simulink subsystem "Human_Input_Pre_Processing"  (R2023b)
settings: Solver=VariableStepAuto  StartTime=0.0  StopTime=10.0  RelTol=1e-3
undefined symbols (not defined in the file): Gamepad_Stick_Neg_Threshold, Gamepad_Stick_Pos_Threshold, Test_DC_Gain_BackLower, Test_DC_Gain_BackUpper, Test_DC_Gain_BallScrew, Test_DC_Gain_Front, Test_DC_Gain_Intake, Test_DC_Gain_Shooter
libraries: simulink x28
settings Model: Creator=ander  LastModifiedBy=ander

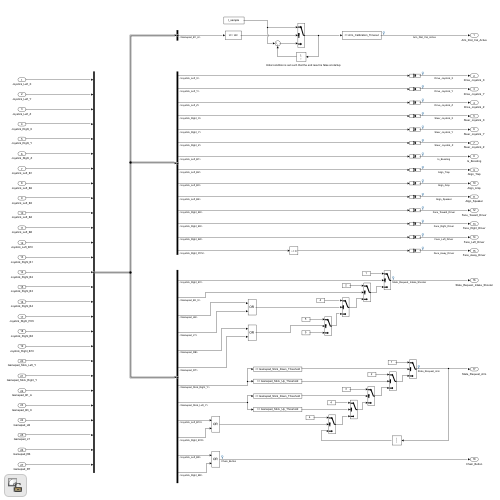
[thumbnail: Simulink's stored preview of the top-level diagram]
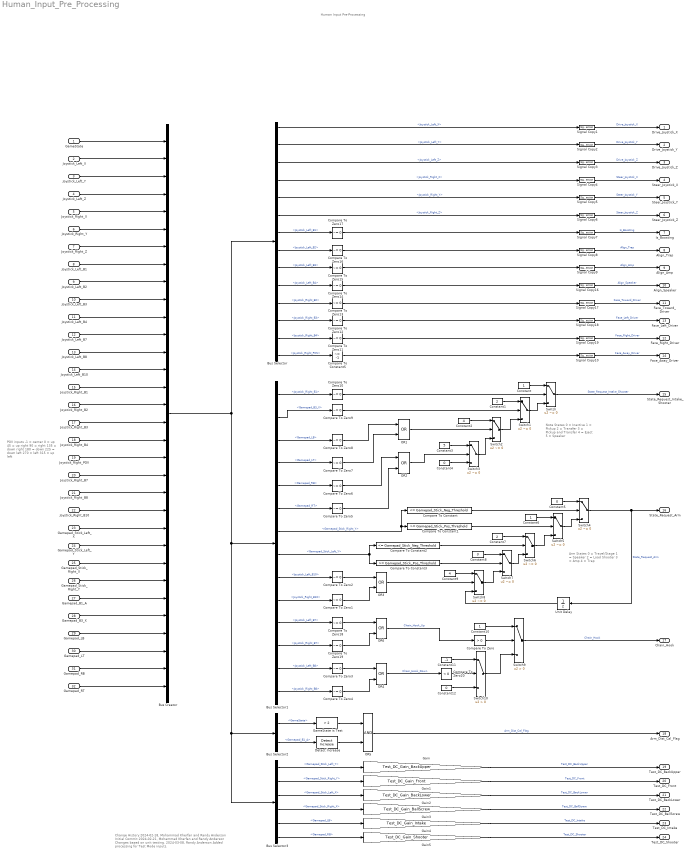
== system Human_Input_Pre_Processing ==
  note: POV inputs
      | -1 = center
      | 0 = up
      | 45 = up right
      | 90 = right
      | 135 = down right
      | 180 = down
      | 225 = down left
      | 270 = left
      | 315 = up left
  note: Human Input Pre-Processing
  note: Change History
      | 2024-02-18, Mohammad Kherfan and Randy Anderson
      | Initial Commit
      | 2024-02-21, Mohammad Kherfan and Randy Anderson
      | Changes based on unit testing.
      | 2024-03-08, Randy Anderson
      | Added processing for Test Mode inputs.
  note: Arm States
      | 0 = Travel/Stage
      | 1 = Speaker
      | 2 = Load Shooter
      | 3 = Amp
      | 4 = Trap
  note: Note States
      | 0 = Inactive
      | 1 = Pickup
      | 2 = Transfer
      | 3 = Pickup and Transfer
      | 4 = Eject
      | 5 = Speaker
  GameState : Inport
  Joystick_Left_X : Inport  Port=2
  Joystick_Left_Y : Inport  Port=3
  Joystick_Left_Z : Inport  Port=4
  Joystick_Right_X : Inport  Port=5
  Joystick_Right_Y : Inport  Port=6
  Joystick_Right_Z : Inport  Port=7
  Joystick_Left_B1 : Inport  Port=8
  Joystick_Left_B2 : Inport  Port=9
  Joystick_Left_B3 : Inport  Port=10
  Joystick_Left_B4 : Inport  Port=11
  Joystick_Left_B7 : Inport  Port=12
  Joystick_Left_B8 : Inport  Port=13
  Joystick_Left_B10 : Inport  Port=14
  Joystick_Right_B1 : Inport  Port=15
  Joystick_Right_B2 : Inport  Port=16
  Joystick_Right_B3 : Inport  Port=17
  Joystick_Right_B4 : Inport  Port=18
  Joystick_Right_POV : Inport  Port=19
  Joystick_Right_B7 : Inport  Port=20
  Joystick_Right_B8 : Inport  Port=21
  Joystick_Right_B10 : Inport  Port=22
  Gamepad_Stick_Left_X : Inport  Port=23
  Gamepad_Stick_Left_Y : Inport  Port=24
  Gamepad_Stick_Right_X : Inport  Port=25
  Gamepad_Stick_Right_Y : Inport  Port=26
  Gamepad_B1_A : Inport  Port=27
  Gamepad_B3_X : Inport  Port=28
  Gamepad_LB : Inport  Port=29
  Gamepad_LT : Inport  Port=30
  Gamepad_RB : Inport  Port=31
  Gamepad_RT : Inport  Port=32
  Bus Creator : BusCreator  Inputs=32
  Bus Selector : BusSelector  OutputSignals=Joystick_Left_X,Joystick_Left_Y,Joystick_Left_Z,Joystick_Right_X,Joystick_Right_Y,Joystick_Right_Z,Joystick_Left_B1,Joystick_Left_B2,Joystick_Left_B3,Joystick_Left_B4,Joystick_Right_B2,Joystick_Right_B3,Joystick_Right_B4,Joystick_Right_POV
  Bus Selector1 : BusSelector  OutputSignals=Joystick_Right_B1,Gamepad_B3_X,Gamepad_LB,Gamepad_LT,Gamepad_RB,Gamepad_RT,Gamepad_Stick_Right_Y,Gamepad_Stick_Left_Y,Joystick_Left_B10,Joystick_Right_B10,Joystick_Left_B7,Joystick_Right_B7,Joystick_Left_B8,Joystick_Right_B8
  Bus Selector2 : BusSelector  OutputSignals=GameState,Gamepad_B1_A
  Bus Selector3 : BusSelector  OutputSignals=Gamepad_Stick_Left_Y,Gamepad_Stick_Right_Y,Gamepad_Stick_Left_X,Gamepad_Stick_Right_X,Gamepad_LB,Gamepad_RB
  Compare To Constant : simulink/Logic and Bit Operations/Compare To Constant  relop=<=  const=Gamepad_Stick_Neg_Threshold  OutDataTypeStr=boolean
  Compare To Constant1 : simulink/Logic and Bit Operations/Compare To Constant  relop=>=  const=Gamepad_Stick_Pos_Threshold  OutDataTypeStr=boolean
  Compare To Constant2 : simulink/Logic and Bit Operations/Compare To Constant  relop=<=  const=Gamepad_Stick_Neg_Threshold  OutDataTypeStr=boolean
  Compare To Constant3 : simulink/Logic and Bit Operations/Compare To Constant  relop=>=  const=Gamepad_Stick_Pos_Threshold  OutDataTypeStr=boolean
  Compare To Constant5 : simulink/Logic and Bit Operations/Compare To Constant  relop=~=  const=-1  OutDataTypeStr=boolean
  Compare To Zero : simulink/Logic and Bit Operations/Compare To Zero  relop=>  OutDataTypeStr=boolean
  Compare To Zero{1..19} (19 alike) : simulink/Logic and Bit Operations/Compare To Zero  relop=~=  OutDataTypeStr=boolean
  Compare To Zero20 : simulink/Logic and Bit Operations/Compare To Zero  relop=<  OutDataTypeStr=boolean
  Constant : Constant
  Constant1 : Constant  Value=2
  Constant10 : Constant
  Constant11 : Constant  Value=-1
  Constant12 : Constant  Value=0
  Constant2 : Constant  Value=4
  Constant3 : Constant  Value=5
  Constant4 : Constant  Value=0
  Constant5 : Constant  Value=0
  Constant6 : Constant
  Constant7 : Constant  Value=2
  Constant8 : Constant  Value=3
  Constant9 : Constant  Value=4
  Detect Increase : simulink/Logic and Bit Operations/Detect Increase  vinit=0.0  OutDataTypeStr=boolean
  Gain : Gain  Gain=Test_DC_Gain_BackUpper
  Gain1 : Gain  Gain=Test_DC_Gain_Front
  Gain2 : Gain  Gain=Test_DC_Gain_BackLower
  Gain3 : Gain  Gain=Test_DC_Gain_BallScrew
  Gain4 : Gain  Gain=Test_DC_Gain_Intake
  Gain5 : Gain  Gain=Test_DC_Gain_Shooter
  GameState is Test : simulink/Logic and Bit Operations/Compare To Constant  relop=>  const=2  OutDataTypeStr=boolean
  OR{1..4,6} (5 alike) : Logic  Operator=OR  AllPortsSameDT=off  OutDataTypeStr=boolean
  OR5 : Logic  AllPortsSameDT=off  OutDataTypeStr=boolean
  Signal Copy{1..10,16..19} (14 alike) : SignalConversion  OverrideOpt=off
  Switch{,1..8} (9 alike) : Switch  Criteria=u2 ~= 0  SaturateOnIntegerOverflow=off  InputSameDT=off
  Switch10 : Switch  Criteria=u2 > Threshold  SaturateOnIntegerOverflow=off  InputSameDT=off
  Switch9 : Switch  Criteria=u2 > Threshold  SaturateOnIntegerOverflow=off  InputSameDT=off
  Unit Delay : UnitDelay  SampleTime=-1  HasFrameUpgradeWarning=on
  Drive_Joystick_X : Outport
  Drive_Joystick_Y : Outport  Port=2
  Drive_Joystick_Z : Outport  Port=3
  Steer_Joystick_X : Outport  Port=4
  Steer_Joystick_Y : Outport  Port=5
  Steer_Joystick_Z : Outport  Port=6
  Is_Boosting : Outport  Port=7
  Align_Trap : Outport  Port=8
  Align_Amp : Outport  Port=9
  Align_Speaker : Outport  Port=10
  Face_Toward_Driver : Outport  Port=11
  Face_Right_Driver : Outport  Port=12
  Face_Left_Driver : Outport  Port=13
  Face_Away_Driver : Outport  Port=14
  State_Request_Intake_Shooter : Outport  Port=15
  State_Request_Arm : Outport  Port=16
  Chain_Hook : Outport  Port=17
  Arm_Dist_Cal_Flag : Outport  Port=18
  Test_DC_BackUpper : Outport  Port=19
  Test_DC_Front : Outport  Port=20
  Test_DC_BackLower : Outport  Port=21
  Test_DC_BallScrew : Outport  Port=22
  Test_DC_Intake : Outport  Port=23
  Test_DC_Shooter : Outport  Port=24
  wires:
  Joystick_Right_Z/1 -> Bus Creator/7
  Joystick_Left_B1/1 -> Bus Creator/8
  Joystick_Left_B2/1 -> Bus Creator/9
  Joystick_Left_B3/1 -> Bus Creator/10
  Joystick_Left_B4/1 -> Bus Creator/11
  Joystick_Left_B8/1 -> Bus Creator/13
  Joystick_Left_B10/1 -> Bus Creator/14
  Joystick_Right_B1/1 -> Bus Creator/15
  Joystick_Right_B2/1 -> Bus Creator/16
  Joystick_Right_B3/1 -> Bus Creator/17
  Joystick_Right_B4/1 -> Bus Creator/18
  Bus Creator/1 -> Bus Selector1/1, Bus Selector2/1, Bus Selector3/1, Bus Selector/1
  Joystick_Left_X/1 -> Bus Creator/2
  Joystick_Left_Y/1 -> Bus Creator/3
  Joystick_Left_Z/1 -> Bus Creator/4
  Joystick_Right_X/1 -> Bus Creator/5
  Joystick_Right_Y/1 -> Bus Creator/6
  Bus Selector/1 -> Signal Copy1/1  "<Joystick_Left_X>"
  Bus Selector/2 -> Signal Copy2/1  "<Joystick_Left_Y>"
  Bus Selector/3 -> Signal Copy3/1  "<Joystick_Left_Z>"
  Bus Selector/4 -> Signal Copy4/1  "<Joystick_Right_X>"
  Bus Selector/5 -> Signal Copy5/1  "<Joystick_Right_Y>"
  Bus Selector/6 -> Signal Copy6/1  "<Joystick_Right_Z>"
  Bus Selector/7 -> Compare To Zero17/1  "<Joystick_Left_B1>"
  Signal Copy1/1 -> Drive_Joystick_X/1  "Drive_Joystick_X"
  Signal Copy7/1 -> Is_Boosting/1  "Is_Boosting"
  Signal Copy6/1 -> Steer_Joystick_Z/1  "Steer_Joystick_Z"
  Signal Copy5/1 -> Steer_Joystick_Y/1  "Steer_Joystick_Y"
  Signal Copy4/1 -> Steer_Joystick_X/1  "Steer_Joystick_X"
  Signal Copy3/1 -> Drive_Joystick_Z/1  "Drive_Joystick_Z"
  Signal Copy2/1 -> Drive_Joystick_Y/1  "Drive_Joystick_Y"
  Bus Selector1/3 -> Compare To Zero8/1  "<Gamepad_LB>"
  Bus Selector1/4 -> Compare To Zero7/1  "<Gamepad_LT>"
  Bus Selector1/5 -> Compare To Zero6/1  "<Gamepad_RB>"
  Bus Selector1/6 -> Compare To Zero5/1  "<Gamepad_RT>"
  Bus Selector1/7 -> Compare To Constant1/1, Compare To Constant/1  "<Gamepad_Stick_Right_Y>"
  Bus Selector1/8 -> Compare To Constant3/1, Compare To Constant2/1  "<Gamepad_Stick_Left_Y>"
  Bus Selector1/9 -> Compare To Zero2/1  "<Joystick_Left_B10>"
  Bus Selector1/10 -> Compare To Zero1/1  "<Joystick_Right_B10>"
  Bus Selector1/13 -> Compare To Zero3/1  "<Joystick_Left_B8>"
  Bus Selector1/14 -> Compare To Zero4/1  "<Joystick_Right_B8>"
  Bus Selector1/1 -> Compare To Zero10/1  "<Joystick_Right_B1>"
  Bus Selector1/2 -> Compare To Zero9/1  "<Gamepad_B3_X>"
  Constant/1 -> Switch/1
  Gamepad_Stick_Left_Y/1 -> Bus Creator/24
  Joystick_Right_B10/1 -> Bus Creator/22
  Gamepad_Stick_Right_Y/1 -> Bus Creator/26
  Joystick_Right_B8/1 -> Bus Creator/21
  Gamepad_B1_A/1 -> Bus Creator/27
  Joystick_Right_POV/1 -> Bus Creator/19
  Gamepad_LB/1 -> Bus Creator/29
  Gamepad_LT/1 -> Bus Creator/30
  Gamepad_RB/1 -> Bus Creator/31
  Gamepad_RT/1 -> Bus Creator/32
  Switch1/1 -> Switch/3
  Switch2/1 -> Switch1/3
  OR1/1 -> Switch2/2
  OR2/1 -> Switch3/2
  Constant2/1 -> Switch2/1
  Constant1/1 -> Switch1/1
  Constant3/1 -> Switch3/1
  Constant4/1 -> Switch3/3
  Switch3/1 -> Switch2/3
  Switch/1 -> State_Request_Intake_Shooter/1  "State_Request_Intake_Shooter"
  Switch7/1 -> Switch6/3
  Switch5/1 -> Switch4/3
  Constant8/1 -> Switch7/1
  Switch6/1 -> Switch5/3
  Constant7/1 -> Switch6/1
  Constant5/1 -> Switch4/1
  Constant6/1 -> Switch5/1
  Compare To Constant/1 -> Switch4/2
  Compare To Constant1/1 -> Switch5/2
  Compare To Constant2/1 -> Switch6/2
  Compare To Constant3/1 -> Switch7/2
  Switch8/1 -> Switch7/3
  Constant9/1 -> Switch8/1
  OR3/1 -> Switch8/2
  Switch4/1 -> Unit Delay/1, State_Request_Arm/1  "State_Request_Arm"
  Signal Copy8/1 -> Align_Trap/1  "Align_Trap"
  Signal Copy9/1 -> Align_Amp/1  "Align_Amp"
  Signal Copy16/1 -> Align_Speaker/1  "Align_Speaker"
  Signal Copy17/1 -> Face_Toward_Driver/1  "Face_Toward_Driver"
  Signal Copy19/1 -> Face_Right_Driver/1  "Face_Right_Driver"
  Signal Copy18/1 -> Face_Left_Driver/1  "Face_Left_Driver"
  Bus Selector/8 -> Compare To Zero16/1  "<Joystick_Left_B2>"
  Bus Selector/9 -> Compare To Zero15/1  "<Joystick_Left_B3>"
  Bus Selector/10 -> Compare To Zero14/1  "<Joystick_Left_B4>"
  Signal Copy10/1 -> Face_Away_Driver/1  "Face_Away_Driver"
  Bus Selector/11 -> Compare To Zero13/1  "<Joystick_Right_B2>"
  Bus Selector/12 -> Compare To Zero12/1  "<Joystick_Right_B3>"
  Bus Selector/13 -> Compare To Zero11/1  "<Joystick_Right_B4>"
  Bus Selector/14 -> Compare To Constant5/1  "<Joystick_Right_POV>"
  Unit Delay/1 -> Switch8/3
  Gamepad_B3_X/1 -> Bus Creator/28
  Bus Selector2/2 -> Detect Increase/1  "<Gamepad_B1_A>"
  OR5/1 -> Arm_Dist_Cal_Flag/1  "Arm_Dist_Cal_Flag"
  Compare To Zero1/1 -> OR3/2
  Compare To Zero2/1 -> OR3/1
  Compare To Zero3/1 -> OR4/1
  Compare To Zero4/1 -> OR4/2
  Compare To Zero5/1 -> OR2/2
  Compare To Zero6/1 -> OR2/1
  Compare To Zero7/1 -> OR1/2
  Compare To Zero8/1 -> OR1/1
  Compare To Zero9/1 -> Switch1/2
  Compare To Zero10/1 -> Switch/2
  Compare To Zero11/1 -> Signal Copy19/1
  Compare To Zero12/1 -> Signal Copy18/1
  Compare To Zero13/1 -> Signal Copy17/1
  Compare To Zero14/1 -> Signal Copy16/1
  Compare To Zero15/1 -> Signal Copy9/1
  Compare To Zero16/1 -> Signal Copy8/1
  Compare To Zero17/1 -> Signal Copy7/1
  Compare To Constant5/1 -> Signal Copy10/1
  GameState/1 -> Bus Creator/1
  Bus Selector2/1 -> GameState is Test/1  "<GameState>"
  GameState is Test/1 -> OR5/1
  Detect Increase/1 -> OR5/2
  Gain/1 -> Test_DC_BackUpper/1  "Test_DC_BackUpper"
  Bus Selector3/5 -> Gain4/1  "<Gamepad_LB>"
  Bus Selector3/6 -> Gain5/1  "<Gamepad_RB>"
  Gain1/1 -> Test_DC_Front/1  "Test_DC_Front"
  Gain2/1 -> Test_DC_BackLower/1  "Test_DC_BackLower"
  Gain3/1 -> Test_DC_BallScrew/1  "Test_DC_BallScrew"
  Gain4/1 -> Test_DC_Intake/1  "Test_DC_Intake"
  Gain5/1 -> Test_DC_Shooter/1  "Test_DC_Shooter"
  Gamepad_Stick_Left_X/1 -> Bus Creator/23
  Gamepad_Stick_Right_X/1 -> Bus Creator/25
  Bus Selector3/1 -> Gain/1  "<Gamepad_Stick_Left_Y>"
  Bus Selector3/2 -> Gain1/1  "<Gamepad_Stick_Right_Y>"
  Bus Selector3/3 -> Gain2/1  "<Gamepad_Stick_Left_X>"
  Bus Selector3/4 -> Gain3/1  "<Gamepad_Stick_Right_X>"
  Joystick_Left_B7/1 -> Bus Creator/12
  Joystick_Right_B7/1 -> Bus Creator/20
  Compare To Zero19/1 -> OR6/2
  Compare To Zero18/1 -> OR6/1
  Bus Selector1/11 -> Compare To Zero18/1  "<Joystick_Left_B7>"
  Bus Selector1/12 -> Compare To Zero19/1  "<Joystick_Right_B7>"
  OR6/1 -> Compare To Zero/1  "Chain_Hook_Up"
  Compare To Zero/1 -> Switch9/2
  Constant10/1 -> Switch9/1
  Switch10/1 -> Switch9/3
  OR4/1 -> Compare To Zero20/1  "Chain_Hook_Down"
  Compare To Zero20/1 -> Switch10/2
  Constant11/1 -> Switch10/1
  Constant12/1 -> Switch10/3
  Switch9/1 -> Chain_Hook/1  "Chain_Hook"
